simulink library "vehicle_model"  (R2020b)
settings: Solver=ode45  StartTime=0.0  StopTime=10.0  RelTol=1e-3  EnableMultiTasking=on
undefined symbols (not defined in the file): DiscIntNeverNeededParam, par_VEH, select_To_Wks_akt, stepsize, v0
libraries: $bdroot x8, pacejka_trans x6, simulink x4, body_chassis_vert x1
(part 3 of 4)

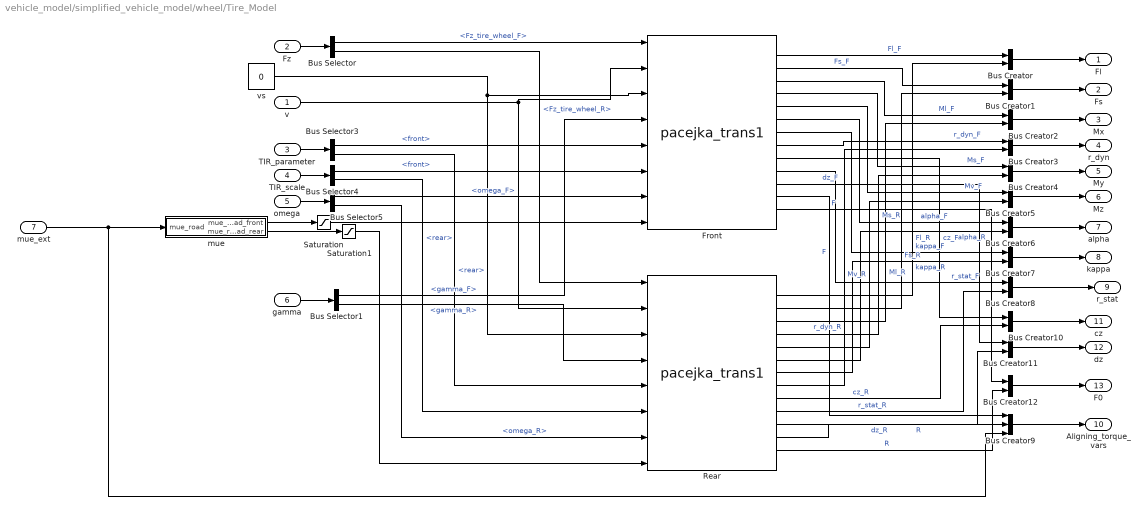
== system vehicle_model/simplified_vehicle_model/wheel/Tire_Model ==
  v : Inport
  Fz : Inport  Port=2
  TIR_parameter : Inport  Port=3
  TIR_scale : Inport  Port=4
  omega : Inport  Port=5
  gamma : Inport  Port=6
  mue_ext : Inport  Port=7
  Bus Creator{,1..8,10..12} (12 alike) : BusCreator  Inputs=2
  Bus Creator9 : BusCreator  Inputs=3
  Bus Selector : BusSelector  OutputSignals=Fz_tire_wheel_F,Fz_tire_wheel_R
  Bus Selector1 : BusSelector  OutputSignals=gamma_F,gamma_R
  Bus Selector3 : BusSelector  OutputSignals=front,rear
  Bus Selector4 : BusSelector  OutputSignals=front,rear
  Bus Selector5 : BusSelector  OutputSignals=omega_F,omega_R
  Front : pacejka_trans/pacejka_trans1  mounted_side_input=right
  Rear : pacejka_trans/pacejka_trans1  mounted_side_input=right
  Saturation : Saturate  UpperLimit=2  LowerLimit=0.05
  Saturation1 : Saturate  UpperLimit=2  LowerLimit=0.05
  mue : Subsystem
  vs : Constant  Value=0
  Fl : Outport  VectorParamsAs1DForOutWhenUnconnected=off
  Fs : Outport  Port=2  VectorParamsAs1DForOutWhenUnconnected=off
  Mx : Outport  Port=3  VectorParamsAs1DForOutWhenUnconnected=off
  r_dyn : Outport  Port=4  VectorParamsAs1DForOutWhenUnconnected=off
  My : Outport  Port=5  VectorParamsAs1DForOutWhenUnconnected=off
  Mz : Outport  Port=6  VectorParamsAs1DForOutWhenUnconnected=off
  alpha : Outport  Port=7  VectorParamsAs1DForOutWhenUnconnected=off
  kappa : Outport  Port=8  VectorParamsAs1DForOutWhenUnconnected=off
  r_stat : Outport  Port=9  VectorParamsAs1DForOutWhenUnconnected=off
  Aligning_torque_vars : Outport  Port=10  VectorParamsAs1DForOutWhenUnconnected=off
  cz : Outport  Port=11  VectorParamsAs1DForOutWhenUnconnected=off
  dz : Outport  Port=12  VectorParamsAs1DForOutWhenUnconnected=off
  F0 : Outport  Port=13  VectorParamsAs1DForOutWhenUnconnected=off
  wires:
  Front/10 -> Bus Creator8/1  "r_stat_F"
  Rear/3 -> Bus Creator2/2  "Ml_R"
  Front/8 -> Bus Creator3/1  "r_dyn_F"
  Rear/10 -> Bus Creator8/2  "r_stat_R"
  Front/5 -> Bus Creator5/1  "Mv_F"
  Bus Selector/2 -> Rear/1  "<Fz_tire_wheel_R>"
  Saturation1/1 -> Rear/8
  Bus Selector/1 -> Front/1  "<Fz_tire_wheel_F>"
  TIR_parameter/1 -> Bus Selector3/1
  Bus Selector4/1 -> Front/6  "<front>"
  Front/1 -> Bus Creator/1  "Fl_F"
  Saturation/1 -> Front/8
  Fz/1 -> Bus Selector/1
  Bus Selector4/2 -> Rear/6  "<rear>"
  Bus Selector1/1 -> Front/4  "<gamma_F>"
  Bus Selector3/1 -> Front/5  "<front>"
  omega/1 -> Bus Selector5/1
  TIR_scale/1 -> Bus Selector4/1
  Bus Selector3/2 -> Rear/5  "<rear>"
  Bus Selector5/1 -> Front/7  "<omega_F>"
  Bus Selector5/2 -> Rear/7  "<omega_R>"
  mue_ext/1 -> Bus Creator9/3, mue/1("mue_road ")
  Bus Creator1/1 -> Fs/1
  Bus Creator2/1 -> Mx/1
  Bus Creator5/1 -> Mz/1
  Rear/2 -> Bus Creator1/2  "Fs_R"
  Bus Creator12/1 -> F0/1
  Bus Creator9/1 -> Aligning_torque_vars/1
  Bus Creator/1 -> Fl/1
  Front/2 -> Bus Creator1/1  "Fs_F"
  Bus Creator6/1 -> alpha/1
  Bus Creator3/1 -> r_dyn/1
  Bus Creator7/1 -> kappa/1
  Bus Creator4/1 -> My/1
  Rear/1 -> Bus Creator/2  "Fl_R"
  Bus Creator11/1 -> dz/1
  Bus Creator10/1 -> cz/1
  Bus Creator8/1 -> r_stat/1
  Rear/9 -> Bus Creator10/2  "cz_R"
  Front/3 -> Bus Creator2/1  "Ml_F"
  Front/7 -> Bus Creator7/1  "kappa_F"
  Rear/8 -> Bus Creator3/2  "r_dyn_R"
  Rear/11 -> Bus Creator11/2  "dz_R"
  Front/11 -> Bus Creator11/1  "dz_F"
  Rear/12 -> Bus Creator9/2  "R"
  Front/13 -> Bus Creator12/1  "F"
  Front/6 -> Bus Creator6/1  "alpha_F"
  Front/12 -> Bus Creator9/1  "F"
  Front/4 -> Bus Creator4/1  "Ms_F"
  Rear/5 -> Bus Creator5/2  "Mv_R"
  Rear/6 -> Bus Creator6/2  "alpha_R"
  Rear/4 -> Bus Creator4/2  "Ms_R"
  Rear/13 -> Bus Creator12/2  "R"
  Front/9 -> Bus Creator10/1  "cz_F"
  Rear/7 -> Bus Creator7/2  "kappa_R"
  vs/1 -> Front/3, Rear/3
  v/1 -> Rear/2, Front/2
  mue/1(mue_road_front) -> Saturation/1
  mue/2(mue_road_rear) -> Saturation1/1
  gamma/1 -> Bus Selector1/1
  Bus Selector1/2 -> Rear/4  "<gamma_R>"

== system vehicle_model/simplified_vehicle_model/wheel/calc_Fz ==
  cz : Inport
  dz : Inport  Port=2
  zwheel : Inport  Port=3
  Bus Creator1 : BusCreator  Inputs=2
  Bus Selector1 : BusSelector  OutputSignals=cz_F,cz_R
  Bus Selector3 : BusSelector  OutputSignals=zwheel_F.zwheel,zwheel_R.zwheel
  Bus Selector4 : BusSelector  OutputSignals=zwheel_F.zwheelp,zwheel_R.zwheelp
  Bus Selector5 : BusSelector  OutputSignals=dz_F,dz_R
  Gain : Gain  Gain=-1
  Gain1 : Gain
  Gain2 : Gain  Gain=-1
  Gain5 : Gain
  Product{,1,4..5} (4 alike) : Product  RndMeth=Zero
  Sum4 : Sum  Inputs=|+-
  Sum5 : Sum  Inputs=|+-
  Fztire : Outport  VectorParamsAs1DForOutWhenUnconnected=off
  wires:
  Gain1/1 -> Product5/2
  Gain5/1 -> Product4/2
  Bus Selector5/2 -> Gain1/1  "<dz_R>"
  Bus Selector5/1 -> Gain5/1  "<dz_F>"
  dz/1 -> Bus Selector5/1
  Product5/1 -> Sum5/2
  Product4/1 -> Sum4/2
  Bus Selector4/1 -> Product4/1  "<zwheelp>"
  Bus Selector4/2 -> Product5/1  "<zwheelp>"
  Sum5/1 -> Bus Creator1/2  "Fz_tire_wheel_R"
  Sum4/1 -> Bus Creator1/1  "Fz_tire_wheel_F"
  Product/1 -> Sum4/1  "Fz_tire_wheel_F"
  Product1/1 -> Sum5/1  "Fz_tire_wheel_R"
  Bus Selector3/2 -> Gain2/1  "<zwheel>"
  Bus Selector3/1 -> Gain/1  "<zwheel>"
  zwheel/1 -> Bus Selector4/1, Bus Selector3/1
  Bus Creator1/1 -> Fztire/1
  Bus Selector1/2 -> Product1/1  "<cz_R>"
  cz/1 -> Bus Selector1/1
  Bus Selector1/1 -> Product/1  "<cz_F>"
  Gain/1 -> Product/2
  Gain2/1 -> Product1/2

== system vehicle_model/simplified_vehicle_model/wheel/calc_omega ==
  M_antr : Inport
  M_brems : Inport  Port=2
  r_dyn : Inport  Port=3
  My : Inport  Port=4
  Fl : Inport  Port=5
  r_stat : Inport  Port=6
  Add : Sum  Inputs=++--
  Add1 : Sum  Inputs=++--
  Add{2..7} (6 alike) : Sum
  Bus Creator : BusCreator  Inputs=2
  Bus Selector2 : BusSelector  OutputSignals=r_stat_F,r_stat_R
  Bus Selector3 : BusSelector  OutputSignals=Ms_F,Ms_R
  Bus Selector4 : BusSelector  OutputSignals=Fl_F,Fl_R
  Bus Selector6 : BusSelector  OutputSignals=r_dyn_F,r_dyn_R
  Bus Selector7 : BusSelector  OutputSignals=M_antr_RF,M_antr_LF,M_antr_RR,M_antr_LR
  Bus Selector8 : BusSelector  OutputSignals=M_brems_RF,M_brems_LF,M_brems_RR,M_brems_LR
  Constant : Constant  Value=v0
  Discrete-Time Integrator1 : DiscreteIntegrator  ExternalReset=sampled level  InitialConditionSource=external  InitialCondition=v0/0.3  SampleTime=-1  ICPrevOutput=DiscIntNeverNeededParam  ICPrevScaledInput=DiscIntNeverNeededParam
  Discrete-Time Integrator2 : DiscreteIntegrator  ExternalReset=sampled level  InitialConditionSource=external  InitialCondition=v0/0.3  SampleTime=-1  ICPrevOutput=DiscIntNeverNeededParam  ICPrevScaledInput=DiscIntNeverNeededParam
  Divide{,1,4..5} (4 alike) : Product  Inputs=*/
  Gain{,1..3} (4 alike) : Gain  Gain=0.5
  Product4 : Product  RndMeth=Zero
  Product5 : Product  RndMeth=Zero
  Unit Delay1 : UnitDelay  InitialCondition=par_VEH.r_stat0  SampleTime=-1  HasFrameUpgradeWarning=on
  Unit Delay2 : UnitDelay  InitialCondition=par_VEH.r_stat0  SampleTime=-1  HasFrameUpgradeWarning=on
  friction : Subsystem
  omega : Outport  VectorParamsAs1DForOutWhenUnconnected=off
  wires:
  friction/2(M_fric_R) -> Add1/4
  friction/1(M_fric_F) -> Add/4
  Bus Selector6/2 -> Unit Delay2/1  "<r_dyn_R>"
  Bus Selector6/1 -> Unit Delay1/1  "<r_dyn_F>"
  r_dyn/1 -> Bus Selector6/1
  Gain3/1 -> Add5/2  "M_brems_R"
  Gain1/1 -> Add5/1  "M_antr_R"
  Gain2/1 -> Add4/2  "M_brems_F"
  Gain/1 -> Add4/1  "M_antr_F"
  [Iwf] -> Divide/2
  Unit Delay2/1 -> Divide5/2
  Unit Delay1/1 -> Divide4/2
  Divide5/1 -> Discrete-Time Integrator1/3
  Divide4/1 -> Discrete-Time Integrator2/3
  Constant/1 -> Divide5/1, Divide4/1
  Divide1/1 -> Discrete-Time Integrator1/1  "omegap_R"
  Divide/1 -> Discrete-Time Integrator2/1  "omegap_F"
  Bus Selector3/2 -> Add1/1  "<Ms_R>"
  Bus Selector3/1 -> Add/1  "<Ms_F>"
  Fl/1 -> Bus Selector4/1
  My/1 -> Bus Selector3/1
  r_stat/1 -> Bus Selector2/1
  Add/1 -> Divide/1
  Add1/1 -> Divide1/1
  Add4/1 -> Add/2
  Add5/1 -> Add1/2
  Bus Selector4/1 -> Product4/1  "<Fl_F>"
  Bus Selector2/1 -> Product4/2  "<r_stat_F>"
  Bus Selector4/2 -> Product5/1  "<Fl_R>"
  Bus Selector2/2 -> Product5/2  "<r_stat_R>"
  Product4/1 -> Add/3
  Product5/1 -> Add1/3
  Bus Creator/1 -> friction/1(omega), omega/1
  Discrete-Time Integrator2/1 -> Bus Creator/1  "omega_F"
  Discrete-Time Integrator1/1 -> Bus Creator/2  "omega_R"
  [Iwr] -> Divide1/2
  [reset] -> Discrete-Time Integrator2/2, Discrete-Time Integrator1/2
  Bus Selector7/3 -> Add3/1  "<M_antr_RR>"
  Bus Selector8/3 -> Add7/1  "<M_brems_RR>"
  Bus Selector7/4 -> Add3/2  "<M_antr_LR>"
  Bus Selector8/4 -> Add7/2  "<M_brems_LR>"
  Bus Selector7/2 -> Add2/2  "<M_antr_LF>"
  Bus Selector8/1 -> Add6/1  "<M_brems_RF>"
  Bus Selector7/1 -> Add2/1  "<M_antr_RF>"
  M_brems/1 -> Bus Selector8/1
  M_antr/1 -> Bus Selector7/1
  Bus Selector8/2 -> Add6/2  "<M_brems_LF>"
  Add2/1 -> Gain/1
  Add3/1 -> Gain1/1
  Add6/1 -> Gain2/1
  Add7/1 -> Gain3/1

== system vehicle_model/simplified_vehicle_model/wheel/v0_korr ==
  vl : Inport
  r_dyn : Inport  Port=2
  omega : Inport  Port=3
  Bus Creator : BusCreator  Inputs=2
  Bus Selector1 : BusSelector  OutputSignals=r_dyn_F,r_dyn_R
  Bus Selector2 : BusSelector  OutputSignals=omega_F,omega_R
  Subsystem1 : Subsystem
  Subsystem2 : $bdroot/vehicle_model/wheel/v0_korr/Subsystem4  SystemSampleTime=-1  VariantActivationTime=update diagram  Latency=0  AutoFrameSizeCalculation=off
  v_low : Constant  Value=0.01  VectorParams1D=off
  omega_out : Outport  VectorParamsAs1DForOutWhenUnconnected=off
  wires:
  r_dyn/1 -> Bus Selector1/1
  omega/1 -> Bus Selector2/1
  Bus Creator/1 -> omega_out/1
  v_low/1 -> Subsystem1/2(v_low), Subsystem2/2
  Bus Selector1/1 -> Subsystem1/3(r_dyn)  "<r_dyn_F>"
  Bus Selector1/2 -> Subsystem2/3  "<r_dyn_R>"
  Bus Selector2/1 -> Subsystem1/4(omega)  "<omega_F>"
  Bus Selector2/2 -> Subsystem2/4  "<omega_R>"
  Subsystem1/1(omega_out) -> Bus Creator/1  "omega_F"
  Subsystem2/1 -> Bus Creator/2  "omega_R"
  vl/1 -> Subsystem2/1, Subsystem1/1(vl)

== system vehicle_model/simplified_vehicle_model/wheel/wheel_lift ==
  Fz_spring : Inport
  Fz_tire_wheel : Inport  Port=2
  init_pos : Inport  Port=3
  Bus Selector : BusSelector  OutputSignals=Fz_tire_wheel_F,Fz_tire_wheel_R
  Bus Selector1 : BusSelector  OutputSignals=Fz_Front,Fz_Rear
  wheel_lift_F : Subsystem
  wheel_lift_R : Subsystem
  zroad : Subsystem
  zwheel_F : Outport  VectorParamsAs1DForOutWhenUnconnected=off
  zwheel_R : Outport  Port=2  VectorParamsAs1DForOutWhenUnconnected=off
  wires:
  zroad/2(zroad_rear) -> wheel_lift_R/3(z_init_rear)
  zroad/1(zroad_front) -> wheel_lift_F/3(z_init_front)
  init_pos/1 -> zroad/1(init_pos)
  Bus Selector1/1 -> wheel_lift_F/2(Fzt)  "<Fz_Front>"
  Bus Selector1/2 -> wheel_lift_R/2(Fzt)  "<Fz_Rear>"
  Bus Selector/2 -> wheel_lift_R/1(Fz_tire_wheel)  "<Fz_tire_wheel_R>"
  Bus Selector/1 -> wheel_lift_F/1(Fz_tire_wheel)  "<Fz_tire_wheel_F>"
  Fz_spring/1 -> Bus Selector1/1
  wheel_lift_R/1(zwheel_rear) -> zwheel_R/1
  Fz_tire_wheel/1 -> Bus Selector/1
  wheel_lift_F/1(zwheel_front) -> zwheel_F/1

== system vehicle_model/vehicle_model/Transformation/trafo_matrix ==
  psi : Inport
  theta : Inport  Port=2
  phi : Inport  Port=3
  Add{1..4} (4 alike) : Sum
  Matrix Concatenate : Concatenate  NumInputs=3  Mode=Multidimensional array  ConcatenateDimension=2
  Matrix Concatenate1 : Concatenate  NumInputs=3
  Matrix Concatenate2 : Concatenate  NumInputs=3
  Matrix Concatenate3 : Concatenate  NumInputs=3
  Product{,1,3,5..6,8,10..11} (8 alike) : Product
  Product{2,4,7,9} (4 alike) : Product  Inputs=3
  Trigonometric Function : Trigonometry  Operator=cos
  Trigonometric Function2 : Trigonometry  Operator=cos
  Trigonometric Function3 : Trigonometry  Operator=cos
  Trigonometric Function6 : Trigonometry
  Trigonometric Function7 : Trigonometry
  Trigonometric Function8 : Trigonometry
  Unary Minus : UnaryMinus
  Unary Minus1 : UnaryMinus
  Unary Minus2 : UnaryMinus
  OT3 : Outport  VectorParamsAs1DForOutWhenUnconnected=off
  wires:
  Product11/1 -> Matrix Concatenate3/2
  Product1/1 -> Add1/1
  Trigonometric Function8/1 -> Unary Minus2/1, Product9/2, Product7/2, Product4/2, Product2/2
  Product4/1 -> Add2/2
  Matrix Concatenate/1 -> OT3/1
  Add2/1 -> Matrix Concatenate1/3
  Trigonometric Function6/1 -> Product3/2, Product2/3, Product11/2, Product8/2, Product7/3
  Trigonometric Function/1 -> Product/1, Unary Minus1/1, Product6/1, Product4/1, Product2/1
  Trigonometric Function2/1 -> Product/2, Product5/2, Product10/1, Product11/1
  Trigonometric Function7/1 -> Unary Minus/1, Product9/1, Product7/1, Product5/1, Product3/1
  Product/1 -> Matrix Concatenate1/1
  Product5/1 -> Matrix Concatenate2/1
  Unary Minus/1 -> Product1/1
  Product3/1 -> Add2/1
  Trigonometric Function3/1 -> Product1/2, Product4/3, Product6/2, Product9/3, Product10/2
  Add1/1 -> Matrix Concatenate1/2
  Unary Minus1/1 -> Product8/1
  Product7/1 -> Add3/2
  theta/1 -> Trigonometric Function8/1, Trigonometric Function2/1
  psi/1 -> Trigonometric Function/1, Trigonometric Function7/1
  Add3/1 -> Matrix Concatenate2/2
  Product8/1 -> Add4/1
  Product9/1 -> Add4/2
  phi/1 -> Trigonometric Function3/1, Trigonometric Function6/1
  Product6/1 -> Add3/1
  Matrix Concatenate3/1 -> Matrix Concatenate/3
  Matrix Concatenate2/1 -> Matrix Concatenate/2
  Unary Minus2/1 -> Matrix Concatenate3/1
  Product10/1 -> Matrix Concatenate3/3
  Add4/1 -> Matrix Concatenate2/3
  Matrix Concatenate1/1 -> Matrix Concatenate/1
  Product2/1 -> Add1/2

== system vehicle_model/vehicle_model/Transformation/trafo_matrix1 ==
  psi : Inport
  theta : Inport  Port=2
  Constant : Constant  Value=0
  Constant1 : Constant  Value=0
  Constant2 : Constant
  Constant3 : Constant  Value=0
  Matrix Concatenate : Concatenate  NumInputs=3  Mode=Multidimensional array  ConcatenateDimension=2
  Matrix Concatenate1 : Concatenate  NumInputs=3
  Matrix Concatenate2 : Concatenate  NumInputs=3
  Matrix Concatenate3 : Concatenate  NumInputs=3
  Product3 : Product
  Product6 : Product
  Trigonometric Function : Trigonometry  Operator=cos
  Trigonometric Function2 : Trigonometry  Operator=cos
  Trigonometric Function7 : Trigonometry
  Trigonometric Function8 : Trigonometry
  Unary Minus : UnaryMinus
  Unary Minus1 : UnaryMinus
  OTo : Outport  VectorParamsAs1DForOutWhenUnconnected=off
  wires:
  Unary Minus1/1 -> Matrix Concatenate3/3
  Trigonometric Function8/1 -> Unary Minus1/1
  Constant3/1 -> Matrix Concatenate3/2
  Constant2/1 -> Matrix Concatenate3/1
  Constant1/1 -> Matrix Concatenate2/1
  Constant/1 -> Matrix Concatenate1/1
  Matrix Concatenate1/1 -> Matrix Concatenate/1
  Matrix Concatenate2/1 -> Matrix Concatenate/2
  Matrix Concatenate3/1 -> Matrix Concatenate/3
  Product6/1 -> Matrix Concatenate2/3
  psi/1 -> Trigonometric Function7/1, Trigonometric Function/1
  theta/1 -> Trigonometric Function8/1, Trigonometric Function2/1
  Unary Minus/1 -> Matrix Concatenate1/2
  Trigonometric Function7/1 -> Product6/2, Unary Minus/1
  Trigonometric Function2/1 -> Product6/1, Product3/2
  Trigonometric Function/1 -> Matrix Concatenate2/2, Product3/1
  Product3/1 -> Matrix Concatenate1/3
  Matrix Concatenate/1 -> OTo/1

== system vehicle_model/vehicle_model/Transformation1/trafo_matrix ==
  psi : Inport
  theta : Inport  Port=2
  phi : Inport  Port=3
  Add{1..4} (4 alike) : Sum
  Matrix Concatenate : Concatenate  NumInputs=3  Mode=Multidimensional array  ConcatenateDimension=2
  Matrix Concatenate1 : Concatenate  NumInputs=3
  Matrix Concatenate2 : Concatenate  NumInputs=3
  Matrix Concatenate3 : Concatenate  NumInputs=3
  Product{,1..2,5..8,10} (8 alike) : Product
  Product{3..4,9,12} (4 alike) : Product  Inputs=3
  Trigonometric Function : Trigonometry  Operator=cos
  Trigonometric Function2 : Trigonometry  Operator=cos
  Trigonometric Function3 : Trigonometry  Operator=cos
  Trigonometric Function6 : Trigonometry
  Trigonometric Function7 : Trigonometry
  Trigonometric Function8 : Trigonometry
  Unary Minus1 : UnaryMinus
  Unary Minus3 : UnaryMinus
  Unary Minus4 : UnaryMinus
  OT3 : Outport  VectorParamsAs1DForOutWhenUnconnected=off
  wires:
  Product10/1 -> Matrix Concatenate3/3
  Add4/1 -> Matrix Concatenate3/2
  Product9/1 -> Add4/2
  Product8/1 -> Add4/1
  Unary Minus1/1 -> Product8/1
  Add3/1 -> Matrix Concatenate3/1
  Product12/1 -> Add3/2
  Product7/1 -> Add3/1
  Add2/1 -> Matrix Concatenate2/2
  Product4/1 -> Add2/2
  Product5/1 -> Add2/1
  Add1/1 -> Matrix Concatenate2/1
  Product3/1 -> Add1/2
  Product2/1 -> Add1/1
  Unary Minus4/1 -> Product2/1
  Trigonometric Function8/1 -> Unary Minus3/1, Product3/2, Product4/2, Product12/2, Product9/2
  Matrix Concatenate/1 -> OT3/1
  Unary Minus3/1 -> Matrix Concatenate1/3
  Trigonometric Function6/1 -> Product3/3, Product4/3, Product6/2, Product7/2, Product8/2
  Trigonometric Function/1 -> Product/1, Product3/1, Product5/1, Product12/1, Unary Minus1/1
  Trigonometric Function2/1 -> Product/2, Product1/2, Product6/1, Product10/1
  Product/1 -> Matrix Concatenate1/1
  Trigonometric Function7/1 -> Product1/1, Unary Minus4/1, Product4/1, Product7/1, Product9/1
  Trigonometric Function3/1 -> Product2/2, Product5/2, Product12/3, Product9/3, Product10/2
  Product1/1 -> Matrix Concatenate1/2
  theta/1 -> Trigonometric Function2/1, Trigonometric Function8/1
  psi/1 -> Trigonometric Function/1, Trigonometric Function7/1
  phi/1 -> Trigonometric Function3/1, Trigonometric Function6/1
  Product6/1 -> Matrix Concatenate2/3
  Matrix Concatenate3/1 -> Matrix Concatenate/3
  Matrix Concatenate2/1 -> Matrix Concatenate/2
  Matrix Concatenate1/1 -> Matrix Concatenate/1

== system vehicle_model/vehicle_model/calc_init/pitch ==
  init_pos : Inport
  Add : Sum
  Add1 : Sum
  Add2 : Sum  Inputs=+-
  Bus Selector : BusSelector  OutputSignals=zroad_RF0,zroad_LF0,zroad_RR0,zroad_LR0
  Divide : Product  Inputs=*/
  Gain : Gain  Gain=0.5
  Gain1 : Gain  Gain=0.5
  Trigonometric Function : Trigonometry  Operator=atan
  init_theta : Outport  VectorParamsAs1DForOutWhenUnconnected=off
  wires:
  Bus Selector/3 -> Add1/1  "<zroad_RR0>"
  Bus Selector/2 -> Add/2  "<zroad_LF0>"
  init_pos/1 -> Bus Selector/1
  Bus Selector/1 -> Add/1  "<zroad_RF0>"
  Add/1 -> Gain/1
  Add1/1 -> Gain1/1
  Bus Selector/4 -> Add1/2  "<zroad_LR0>"
  Gain/1 -> Add2/1
  Gain1/1 -> Add2/2
  Add2/1 -> Divide/1
  Divide/1 -> Trigonometric Function/1
  [l] -> Divide/2
  Trigonometric Function/1 -> init_theta/1

== system vehicle_model/vehicle_model/calc_init/roll ==
  init_pos : Inport
  Add : Sum
  Add1 : Sum
  Add2 : Sum  Inputs=+-
  Add3 : Sum
  Bus Selector : BusSelector  OutputSignals=zroad_RF0,zroad_RR0,zroad_LF0,zroad_LR0
  Divide : Product  Inputs=*/
  Gain : Gain  Gain=0.5
  Gain1 : Gain  Gain=0.5
  Gain2 : Gain  Gain=0.5
  Trigonometric Function : Trigonometry  Operator=atan
  init_phi : Outport  VectorParamsAs1DForOutWhenUnconnected=off
  wires:
  Trigonometric Function/1 -> init_phi/1
  Gain2/1 -> Divide/2
  Add3/1 -> Gain2/1
  [sR] -> Add3/2
  [sF] -> Add3/1
  Divide/1 -> Trigonometric Function/1
  Add2/1 -> Divide/1
  Gain1/1 -> Add2/2
  Gain/1 -> Add2/1
  Bus Selector/2 -> Add/2  "<zroad_RR0>"
  Bus Selector/4 -> Add1/2  "<zroad_LR0>"
  Add1/1 -> Gain1/1
  Add/1 -> Gain/1
  Bus Selector/3 -> Add1/1  "<zroad_LF0>"
  Bus Selector/1 -> Add/1  "<zroad_RF0>"
  init_pos/1 -> Bus Selector/1

== system vehicle_model/vehicle_model/calc_init/vertical ==
  init_pos : Inport
  theta : Inport  Port=2
  Add : Sum
  Add1 : Sum
  Bus Selector : BusSelector  OutputSignals=zroad_RF0,zroad_LF0
  Gain : Gain  Gain=0.5
  Product : Product  RndMeth=Zero
  Trigonometric Function : Trigonometry
  init_z0 : Outport  VectorParamsAs1DForOutWhenUnconnected=off
  wires:
  Add1/1 -> init_z0/1
  Product/1 -> Add1/2
  Trigonometric Function/1 -> Product/2
  theta/1 -> Trigonometric Function/1
  [lF] -> Product/1
  Gain/1 -> Add1/1
  Add/1 -> Gain/1
  Bus Selector/2 -> Add/2  "<zroad_LF0>"
  Bus Selector/1 -> Add/1  "<zroad_RF0>"
  init_pos/1 -> Bus Selector/1

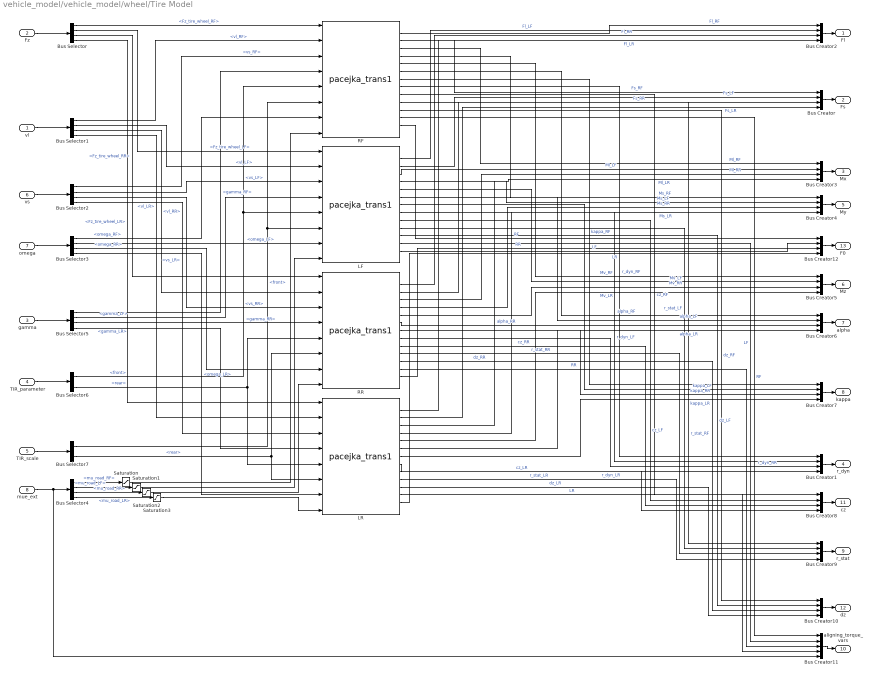
== system vehicle_model/vehicle_model/wheel/Tire Model ==
  vl : Inport
  Fz : Inport  Port=2
  gamma : Inport  Port=3
  TIR_parameter : Inport  Port=4
  TIR_scale : Inport  Port=5
  vs : Inport  Port=6
  omega : Inport  Port=7
  mue_ext : Inport  Port=8
  Bus Creator{,1..10,12} (12 alike) : BusCreator  Inputs=4
  Bus Creator11 : BusCreator  Inputs=5
  Bus Selector : BusSelector  OutputSignals=Fz_tire_wheel_RF,Fz_tire_wheel_LF,Fz_tire_wheel_RR,Fz_tire_wheel_LR
  Bus Selector1 : BusSelector  OutputSignals=vl_RF,vl_LF,vl_RR,vl_LR
  Bus Selector2 : BusSelector  OutputSignals=vs_RF,vs_LF,vs_RR,vs_LR
  Bus Selector3 : BusSelector  OutputSignals=omega_RF,omega_LF,omega_RR,omega_LR
  Bus Selector4 : BusSelector  OutputSignals=mu_road_RF,mu_road_LF,mu_road_RR,mu_road_LR
  Bus Selector5 : BusSelector  OutputSignals=gamma_RF,gamma_LF,gamma_RR,gamma_LR
  Bus Selector6 : BusSelector  OutputSignals=front,rear
  Bus Selector7 : BusSelector  OutputSignals=front,rear
  LF : pacejka_trans/pacejka_trans1  mounted_side_input=left
  LR : pacejka_trans/pacejka_trans1  mounted_side_input=left
  RF : pacejka_trans/pacejka_trans1  mounted_side_input=right
  RR : pacejka_trans/pacejka_trans1  mounted_side_input=right
  Saturation{,1..3} (4 alike) : Saturate  UpperLimit=2  LowerLimit=0.05
  Fl : Outport  VectorParamsAs1DForOutWhenUnconnected=off
  Fs : Outport  Port=2  VectorParamsAs1DForOutWhenUnconnected=off
  Mx : Outport  Port=3  VectorParamsAs1DForOutWhenUnconnected=off
  r_dyn : Outport  Port=4  VectorParamsAs1DForOutWhenUnconnected=off
  My : Outport  Port=5  VectorParamsAs1DForOutWhenUnconnected=off
  Mz : Outport  Port=6  VectorParamsAs1DForOutWhenUnconnected=off
  alpha : Outport  Port=7  VectorParamsAs1DForOutWhenUnconnected=off
  kappa : Outport  Port=8  VectorParamsAs1DForOutWhenUnconnected=off
  r_stat : Outport  Port=9  VectorParamsAs1DForOutWhenUnconnected=off
  aligning_torque_vars : Outport  Port=10  VectorParamsAs1DForOutWhenUnconnected=off
  cz : Outport  Port=11  VectorParamsAs1DForOutWhenUnconnected=off
  dz : Outport  Port=12  VectorParamsAs1DForOutWhenUnconnected=off
  F0 : Outport  Port=13  VectorParamsAs1DForOutWhenUnconnected=off
  wires:
  LR/13 -> Bus Creator12/4  "LR"
  RR/13 -> Bus Creator12/3  "RR"
  LF/13 -> Bus Creator12/2  "LF"
  RF/13 -> Bus Creator12/1  "RF"
  Bus Creator12/1 -> F0/1
  LR/12 -> Bus Creator11/4  "LR"
  RR/12 -> Bus Creator11/3  "RR"
  LF/12 -> Bus Creator11/2  "LF"
  RF/12 -> Bus Creator11/1  "RF"
  Bus Creator11/1 -> aligning_torque_vars/1
  Bus Selector7/2 -> RR/6, LR/6  "<rear>"
  Bus Selector6/2 -> LR/5, RR/5  "<rear>"
  Bus Selector7/1 -> RF/6, LF/6  "<front>"
  Bus Selector6/1 -> LF/5, RF/5  "<front>"
  TIR_scale/1 -> Bus Selector7/1
  TIR_parameter/1 -> Bus Selector6/1
  Saturation3/1 -> LR/8
  Saturation2/1 -> RR/8
  Saturation1/1 -> LF/8
  Saturation/1 -> RF/8
  Bus Selector5/4 -> LR/4  "<gamma_LR>"
  Bus Selector5/3 -> RR/4  "<gamma_RR>"
  Bus Selector5/2 -> LF/4  "<gamma_LF>"
  Bus Selector5/1 -> RF/4  "<gamma_RF>"
  gamma/1 -> Bus Selector5/1
  LR/11 -> Bus Creator10/4  "dz_LR"
  RR/11 -> Bus Creator10/3  "dz_RR"
  LF/11 -> Bus Creator10/2  "dz_LF"
  RF/11 -> Bus Creator10/1  "dz_RF"
  Bus Creator10/1 -> dz/1
  LR/10 -> Bus Creator9/4  "r_stat_LR"
  RR/10 -> Bus Creator9/3  "r_stat_RR"
  LF/10 -> Bus Creator9/2  "r_stat_LF"
  RF/10 -> Bus Creator9/1  "r_stat_RF"
  Bus Creator9/1 -> r_stat/1
  LR/9 -> Bus Creator8/4  "cz_LR"
  RR/9 -> Bus Creator8/3  "cz_RR"
  LF/9 -> Bus Creator8/2  "cz_LF"
  RF/9 -> Bus Creator8/1  "cz_RF"
  Bus Creator8/1 -> cz/1
  Bus Selector4/4 -> Saturation3/1  "<mu_road_LR>"
  Bus Selector4/3 -> Saturation2/1  "<mu_road_RR>"
  Bus Selector4/2 -> Saturation1/1  "<mu_road_LF>"
  Bus Selector4/1 -> Saturation/1  "<mu_road_RF>"
  mue_ext/1 -> Bus Selector4/1, Bus Creator11/5
  Bus Creator/1 -> Fs/1
  RF/2 -> Bus Creator/1  "Fs_RF"
  LF/2 -> Bus Creator/2  "Fs_LF"
  LR/2 -> Bus Creator/4  "Fs_LR"
  RR/2 -> Bus Creator/3  "Fs_RR"
  Bus Creator1/1 -> r_dyn/1
  RF/8 -> Bus Creator1/1  "r_dyn_RF"
  LF/8 -> Bus Creator1/2  "r_dyn_LF"
  RR/8 -> Bus Creator1/3  "r_dyn_RR"
  LR/8 -> Bus Creator1/4  "r_dyn_LR"
  Bus Creator2/1 -> Fl/1
  RF/1 -> Bus Creator2/1  "Fl_RF"
  LF/1 -> Bus Creator2/2  "Fl_LF"
  RR/1 -> Bus Creator2/3  "Fl_RR"
  LR/1 -> Bus Creator2/4  "Fl_LR"
  Bus Creator3/1 -> Mx/1
  Bus Creator4/1 -> My/1
  Bus Creator5/1 -> Mz/1
  Bus Creator6/1 -> alpha/1
  Bus Creator7/1 -> kappa/1
  RF/3 -> Bus Creator3/1  "Ml_RF"
  LF/3 -> Bus Creator3/2  "Ml_LF"
  RR/3 -> Bus Creator3/3  "Ml_RR"
  LR/3 -> Bus Creator3/4  "Ml_LR"
  RF/4 -> Bus Creator4/1  "Ms_RF"
  LF/4 -> Bus Creator4/2  "Ms_LF"
  RR/4 -> Bus Creator4/3  "Ms_RR"
  LR/4 -> Bus Creator4/4  "Ms_LR"
  RF/5 -> Bus Creator5/1  "Mv_RF"
  LF/5 -> Bus Creator5/2  "Mv_LF"
  RR/5 -> Bus Creator5/3  "Mv_RR"
  LR/5 -> Bus Creator5/4  "Mv_LR"
  RF/6 -> Bus Creator6/1  "alpha_RF"
  RR/6 -> Bus Creator6/3  "alpha_RR"
  LF/6 -> Bus Creator6/2  "alpha_LF"
  LR/6 -> Bus Creator6/4  "alpha_LR"
  RF/7 -> Bus Creator7/1  "kappa_RF"
  LF/7 -> Bus Creator7/2  "kappa_LF"
  RR/7 -> Bus Creator7/3  "kappa_RR"
  LR/7 -> Bus Creator7/4  "kappa_LR"
  Fz/1 -> Bus Selector/1
  vl/1 -> Bus Selector1/1
  vs/1 -> Bus Selector2/1
  Bus Selector/1 -> RF/1  "<Fz_tire_wheel_RF>"
  Bus Selector/2 -> LF/1  "<Fz_tire_wheel_LF>"
  Bus Selector/3 -> RR/1  "<Fz_tire_wheel_RR>"
  Bus Selector/4 -> LR/1  "<Fz_tire_wheel_LR>"
  Bus Selector1/1 -> RF/2  "<vl_RF>"
  Bus Selector1/2 -> LF/2  "<vl_LF>"
  Bus Selector1/3 -> RR/2  "<vl_RR>"
  Bus Selector1/4 -> LR/2  "<vl_LR>"
  omega/1 -> Bus Selector3/1
  Bus Selector3/1 -> RF/7  "<omega_RF>"
  Bus Selector3/2 -> LF/7  "<omega_LF>"
  Bus Selector3/3 -> RR/7  "<omega_RR>"
  Bus Selector3/4 -> LR/7  "<omega_LR>"
  Bus Selector2/1 -> RF/3  "<vs_RF>"
  Bus Selector2/2 -> LF/3  "<vs_LF>"
  Bus Selector2/3 -> RR/3  "<vs_RR>"
  Bus Selector2/4 -> LR/3  "<vs_LR>"

== system vehicle_model/vehicle_model/wheel/calc_Fz ==
  cz : Inport
  dz : Inport  Port=2
  zwheel : Inport  Port=3
  Bus Creator : BusCreator  Inputs=4
  Bus Selector : BusSelector  OutputSignals=cz_RF,cz_LF,cz_RR,cz_LR
  Bus Selector2 : BusSelector  OutputSignals=zwheel_RF.zwheel,zwheel_LF.zwheel,zwheel_RR.zwheel,zwheel_LR.zwheel
  Bus Selector3 : BusSelector  OutputSignals=dz_RF,dz_LF,dz_RR,dz_LR
  Bus Selector4 : BusSelector  OutputSignals=zwheel_RF.zwheelp,zwheel_LF.zwheelp,zwheel_RR.zwheelp,zwheel_LR.zwheelp
  Gain{,4,6..7} (4 alike) : Gain  Gain=-1
  Gain{1..3,5} (4 alike) : Gain
  Product{,1..7} (8 alike) : Product  RndMeth=Zero
  Sum{4..7} (4 alike) : Sum  Inputs=|+-
  Fztire : Outport  VectorParamsAs1DForOutWhenUnconnected=off
  wires:
  Bus Selector/1 -> Product/1  "<cz_RF>"
  cz/1 -> Bus Selector/1
  Bus Selector/2 -> Product1/1  "<cz_LF>"
  Bus Creator/1 -> Fztire/1
  zwheel/1 -> Bus Selector2/1, Bus Selector4/1
  Bus Selector2/1 -> Gain4/1  "<zwheel>"
  Bus Selector2/2 -> Gain6/1  "<zwheel>"
  Bus Selector2/3 -> Gain/1  "<zwheel>"
  Bus Selector2/4 -> Gain7/1  "<zwheel>"
  Bus Selector/3 -> Product2/1  "<cz_RR>"
  Bus Selector/4 -> Product3/1  "<cz_LR>"
  Product3/1 -> Sum7/1  "Fz_tire_wheel_LR"
  Product2/1 -> Sum6/1  "Fz_tire_wheel_RR"
  Product1/1 -> Sum5/1  "Fz_tire_wheel_LF"
  Product/1 -> Sum4/1  "Fz_tire_wheel_RF"
  Sum4/1 -> Bus Creator/1  "Fz_tire_wheel_RF"
  Sum5/1 -> Bus Creator/2  "Fz_tire_wheel_LF"
  Sum6/1 -> Bus Creator/3  "Fz_tire_wheel_RR"
  Sum7/1 -> Bus Creator/4  "Fz_tire_wheel_LR"
  Bus Selector4/4 -> Product7/1  "<zwheelp>"
  Bus Selector4/3 -> Product6/1  "<zwheelp>"
  Bus Selector4/2 -> Product5/1  "<zwheelp>"
  Bus Selector4/1 -> Product4/1  "<zwheelp>"
  Product4/1 -> Sum4/2
  Product5/1 -> Sum5/2
  Product6/1 -> Sum6/2
  Product7/1 -> Sum7/2
  dz/1 -> Bus Selector3/1
  Bus Selector3/1 -> Gain5/1  "<dz_RF>"
  Bus Selector3/2 -> Gain1/1  "<dz_LF>"
  Bus Selector3/3 -> Gain2/1  "<dz_RR>"
  Bus Selector3/4 -> Gain3/1  "<dz_LR>"
  Gain5/1 -> Product4/2
  Gain1/1 -> Product5/2
  Gain2/1 -> Product6/2
  Gain3/1 -> Product7/2
  Gain/1 -> Product2/2
  Gain4/1 -> Product/2
  Gain6/1 -> Product1/2
  Gain7/1 -> Product3/2

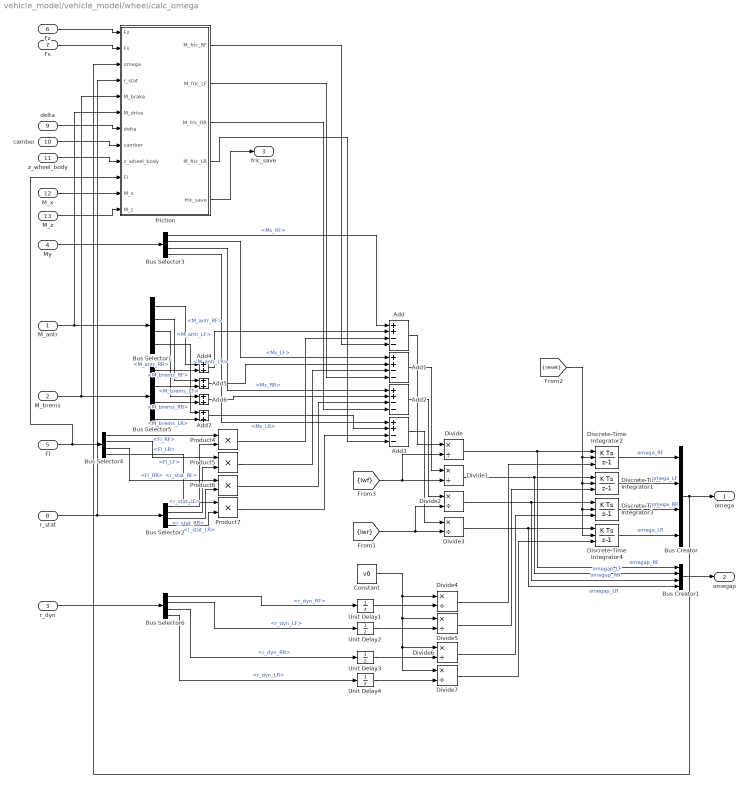
== system vehicle_model/vehicle_model/wheel/calc_omega ==
  M_antr : Inport
  M_brems : Inport  Port=2
  r_dyn : Inport  Port=3
  My : Inport  Port=4
  Fl : Inport  Port=5
  Fz : Inport  Port=6
  Fs : Inport  Port=7
  r_stat : Inport  Port=8
  delta : Inport  Port=9
  camber : Inport  Port=10
  z_wheel_body : Inport  Port=11
  M_x : Inport  Port=12
  M_z : Inport  Port=13
  Add{,1..3} (4 alike) : Sum  Inputs=++--
  Add{4..7} (4 alike) : Sum
  Bus Creator : BusCreator  Inputs=4
  Bus Creator1 : BusCreator  Inputs=4
  Bus Selector1 : BusSelector  OutputSignals=M_antr_RF,M_antr_LF,M_antr_RR,M_antr_LR
  Bus Selector2 : BusSelector  OutputSignals=r_stat_RF,r_stat_LF,r_stat_RR,r_stat_LR
  Bus Selector3 : BusSelector  OutputSignals=Ms_RF,Ms_LF,Ms_RR,Ms_LR
  Bus Selector4 : BusSelector  OutputSignals=Fl_RF,Fl_LF,Fl_RR,Fl_LR
  Bus Selector5 : BusSelector  OutputSignals=M_brems_RF,M_brems_LF,M_brems_RR,M_brems_LR
  Bus Selector6 : BusSelector  OutputSignals=r_dyn_RF,r_dyn_LF,r_dyn_RR,r_dyn_LR
  Constant : Constant  Value=v0
  Discrete-Time Integrator{1..4} (4 alike) : DiscreteIntegrator  ExternalReset=sampled level  InitialConditionSource=external  InitialCondition=v0/0.3  SampleTime=-1  ICPrevOutput=DiscIntNeverNeededParam  ICPrevScaledInput=DiscIntNeverNeededParam
  Divide{,1..7} (8 alike) : Product  Inputs=*/
  Product{4..7} (4 alike) : Product  RndMeth=Zero
  Unit Delay{1..4} (4 alike) : UnitDelay  InitialCondition=par_VEH.r_stat0  SampleTime=-1  HasFrameUpgradeWarning=on
  friction : Subsystem
  omega : Outport  VectorParamsAs1DForOutWhenUnconnected=off
  omegap : Outport  Port=2  VectorParamsAs1DForOutWhenUnconnected=off
  fric_save : Outport  Port=3  VectorParamsAs1DForOutWhenUnconnected=off
  wires:
  [reset] -> Discrete-Time Integrator4/2, Discrete-Time Integrator3/2, Discrete-Time Integrator1/2, Discrete-Time Integrator2/2
  [Iwr] -> Divide2/2, Divide3/2
  Discrete-Time Integrator4/1 -> Bus Creator/4  "omega_LR"
  Discrete-Time Integrator3/1 -> Bus Creator/3  "omega_RR"
  Discrete-Time Integrator1/1 -> Bus Creator/2  "omega_LF"
  Discrete-Time Integrator2/1 -> Bus Creator/1  "omega_RF"
  Bus Creator1/1 -> omegap/1
  Bus Creator/1 -> omega/1, friction/3(omega)
  Product6/1 -> Add2/3
  Product5/1 -> Add1/3
  Product4/1 -> Add/3
  Bus Selector2/4 -> Product7/2  "<r_stat_LR>"
  Bus Selector4/4 -> Product7/1  "<Fl_LR>"
  Bus Selector2/3 -> Product6/2  "<r_stat_RR>"
  Bus Selector4/3 -> Product6/1  "<Fl_RR>"
  Bus Selector2/2 -> Product5/2  "<r_stat_LF>"
  Bus Selector4/2 -> Product5/1  "<Fl_LF>"
  Bus Selector2/1 -> Product4/2  "<r_stat_RF>"
  Bus Selector4/1 -> Product4/1  "<Fl_RF>"
  Add7/1 -> Add3/2
  Add6/1 -> Add2/2
  Add5/1 -> Add1/2
  Add4/1 -> Add/2
  Add3/1 -> Divide3/1
  Add2/1 -> Divide2/1
  Add1/1 -> Divide1/1
  Add/1 -> Divide/1
  r_stat/1 -> Bus Selector2/1, friction/4(r_stat)
  M_antr/1 -> friction/6(M_drive), Bus Selector1/1
  My/1 -> Bus Selector3/1
  Fl/1 -> friction/10(Fl), Bus Selector4/1
  Bus Selector3/1 -> Add/1  "<Ms_RF>"
  Bus Selector3/2 -> Add1/1  "<Ms_LF>"
  Bus Selector3/3 -> Add2/1  "<Ms_RR>"
  Bus Selector3/4 -> Add3/1  "<Ms_LR>"
  Divide/1 -> Bus Creator1/1, Discrete-Time Integrator2/1  "omegap_RF"
  Divide1/1 -> Bus Creator1/2, Discrete-Time Integrator1/1  "omegap_LF"
  Divide2/1 -> Bus Creator1/3, Discrete-Time Integrator3/1  "omegap_RR"
  Divide3/1 -> Bus Creator1/4, Discrete-Time Integrator4/1  "omegap_LR"
  Constant/1 -> Divide4/1, Divide5/1, Divide6/1, Divide7/1
  Divide4/1 -> Discrete-Time Integrator2/3
  Divide5/1 -> Discrete-Time Integrator1/3
  Divide6/1 -> Discrete-Time Integrator3/3
  Divide7/1 -> Discrete-Time Integrator4/3
  Unit Delay1/1 -> Divide4/2
  Unit Delay2/1 -> Divide5/2
  Unit Delay3/1 -> Divide6/2
  Unit Delay4/1 -> Divide7/2
  Product7/1 -> Add3/3
  [Iwf] -> Divide/2, Divide1/2
  M_brems/1 -> friction/5(M_brake), Bus Selector5/1
  Bus Selector1/1 -> Add4/1  "<M_antr_RF>"
  Bus Selector5/1 -> Add4/2  "<M_brems_RF>"
  Bus Selector1/2 -> Add5/1  "<M_antr_LF>"
  Bus Selector5/2 -> Add5/2  "<M_brems_LF>"
  Bus Selector1/3 -> Add6/1  "<M_antr_RR>"
  Bus Selector5/3 -> Add6/2  "<M_brems_RR>"
  Bus Selector1/4 -> Add7/1  "<M_antr_LR>"
  Bus Selector5/4 -> Add7/2  "<M_brems_LR>"
  r_dyn/1 -> Bus Selector6/1
  Bus Selector6/1 -> Unit Delay1/1  "<r_dyn_RF>"
  Bus Selector6/2 -> Unit Delay2/1  "<r_dyn_LF>"
  Bus Selector6/3 -> Unit Delay3/1  "<r_dyn_RR>"
  Bus Selector6/4 -> Unit Delay4/1  "<r_dyn_LR>"
  Fz/1 -> friction/1(Fz)
  Fs/1 -> friction/2(Fs)
  friction/1(M_fric_RF) -> Add/4
  friction/2(M_fric_LF) -> Add1/4
  friction/3(M_fric_RR) -> Add2/4
  friction/4(M_fric_LR) -> Add3/4
  delta/1 -> friction/7(delta)
  camber/1 -> friction/8(camber)
  z_wheel_body/1 -> friction/9(z_wheel_body)
  friction/5(fric_save) -> fric_save/1
  M_x/1 -> friction/11(M_x)
  M_z/1 -> friction/12(M_z)

== system vehicle_model/vehicle_model/wheel/calc_v ==
  delta : Inport
  beta : Inport  Port=2
  psi : Inport  Port=3
  v : Inport  Port=4
  calc_vl : Subsystem
  calc_vs : Subsystem
  vs : Outport  VectorParamsAs1DForOutWhenUnconnected=off
  vl : Outport  Port=2  VectorParamsAs1DForOutWhenUnconnected=off
  wires:
  calc_vs/1(vs) -> vs/1
  beta/1 -> calc_vs/7(beta), calc_vl/7(beta)
  v/1 -> calc_vs/5(v), calc_vl/5(v)
  calc_vl/1(vl) -> vl/1
  [lR] -> calc_vs/2(lR), calc_vl/2(lR)
  [lF] -> calc_vs/1(lF), calc_vl/1(lF)
  [sR05] -> calc_vs/4(sR05), calc_vl/4(sR05)
  [sF05] -> calc_vs/3(sF05), calc_vl/3(sF05)
  delta/1 -> calc_vs/8(delta), calc_vl/8(delta)
  psi/1 -> calc_vs/6(psi), calc_vl/6(psi)
  [ySP] -> calc_vl/9(ySP), calc_vs/9(ySP)

== system vehicle_model/vehicle_model/wheel/v0_korr ==
  vl : Inport
  r_dyn : Inport  Port=2
  omega : Inport  Port=3
  Bus Creator : BusCreator  Inputs=4
  Bus Selector : BusSelector  OutputSignals=vl_RF,vl_LF,vl_RR,vl_LR
  Bus Selector1 : BusSelector  OutputSignals=r_dyn_RF,r_dyn_LF,r_dyn_RR,r_dyn_LR
  Bus Selector2 : BusSelector  OutputSignals=omega_RF,omega_LF,omega_RR,omega_LR
  Subsystem1 : $bdroot/vehicle_model/wheel/v0_korr/Subsystem4  SystemSampleTime=-1  VariantActivationTime=update diagram  Latency=0  AutoFrameSizeCalculation=off
  Subsystem2 : $bdroot/vehicle_model/wheel/v0_korr/Subsystem4  SystemSampleTime=-1  VariantActivationTime=update diagram  Latency=0  AutoFrameSizeCalculation=off
  Subsystem3 : $bdroot/vehicle_model/wheel/v0_korr/Subsystem4  SystemSampleTime=-1  VariantActivationTime=update diagram  Latency=0  AutoFrameSizeCalculation=off
  Subsystem4 : Subsystem
  v_low : Constant  Value=0.01  VectorParams1D=off
  omega_out : Outport  VectorParamsAs1DForOutWhenUnconnected=off
  wires:
  Subsystem3/1 -> Bus Creator/4  "omega_LR"
  Subsystem2/1 -> Bus Creator/3  "omega_RR"
  Subsystem1/1 -> Bus Creator/2  "omega_LF"
  Subsystem4/1(omega_out) -> Bus Creator/1  "omega_RF"
  Bus Selector2/4 -> Subsystem3/4  "<omega_LR>"
  Bus Selector2/3 -> Subsystem2/4  "<omega_RR>"
  Bus Selector2/2 -> Subsystem1/4  "<omega_LF>"
  Bus Selector2/1 -> Subsystem4/4(omega)  "<omega_RF>"
  Bus Selector1/4 -> Subsystem3/3  "<r_dyn_LR>"
  Bus Selector1/3 -> Subsystem2/3  "<r_dyn_RR>"
  Bus Selector1/2 -> Subsystem1/3  "<r_dyn_LF>"
  Bus Selector1/1 -> Subsystem4/3(r_dyn)  "<r_dyn_RF>"
  v_low/1 -> Subsystem1/2, Subsystem2/2, Subsystem3/2, Subsystem4/2(v_low)
  Bus Selector/4 -> Subsystem3/1  "<vl_LR>"
  Bus Selector/3 -> Subsystem2/1  "<vl_RR>"
  Bus Selector/2 -> Subsystem1/1  "<vl_LF>"
  Bus Selector/1 -> Subsystem4/1(vl)  "<vl_RF>"
  Bus Creator/1 -> omega_out/1
  omega/1 -> Bus Selector2/1
  r_dyn/1 -> Bus Selector1/1
  vl/1 -> Bus Selector/1

== system vehicle_model/vehicle_model/wheel/wheel_lift ==
  Fz_spring : Inport
  Fz_tire_wheel : Inport  Port=2
  init_pos : Inport  Port=3
  Bus Selector : BusSelector  OutputSignals=Fz_tire_wheel_RF,Fz_tire_wheel_LF,Fz_tire_wheel_RR,Fz_tire_wheel_LR
  Bus Selector1 : BusSelector  OutputSignals=Fz_RF,Fz_LF,Fz_RR,Fz_LR
  Bus Selector2 : BusSelector  OutputSignals=zroad_RF0,zroad_LF0,zroad_RR0,zroad_LR0
  wheel_lift_LF : $bdroot/vehicle_model/wheel/wheel_lift/wheel_lift_RF  SystemSampleTime=-1  VariantActivationTime=update diagram  Latency=0  AutoFrameSizeCalculation=off
  wheel_lift_LR : $bdroot/vehicle_model/wheel/wheel_lift/wheel_lift_RR  SystemSampleTime=-1  VariantActivationTime=update diagram  Latency=0  AutoFrameSizeCalculation=off
  wheel_lift_RF : Subsystem
  wheel_lift_RR : Subsystem
  zwheel_RF : Outport  VectorParamsAs1DForOutWhenUnconnected=off
  zwheel_LF : Outport  Port=2  VectorParamsAs1DForOutWhenUnconnected=off
  zwheel_RR : Outport  Port=3  VectorParamsAs1DForOutWhenUnconnected=off
  zwheel_LR : Outport  Port=4  VectorParamsAs1DForOutWhenUnconnected=off
  wires:
  wheel_lift_RF/1(zwheel) -> zwheel_RF/1
  Fz_tire_wheel/1 -> Bus Selector/1
  wheel_lift_LF/1 -> zwheel_LF/1
  Fz_spring/1 -> Bus Selector1/1
  wheel_lift_RR/1(zwheel) -> zwheel_RR/1
  wheel_lift_LR/1 -> zwheel_LR/1
  Bus Selector/1 -> wheel_lift_RF/1(Fz_tire_wheel)  "<Fz_tire_wheel_RF>"
  Bus Selector/2 -> wheel_lift_LF/1  "<Fz_tire_wheel_LF>"
  Bus Selector/3 -> wheel_lift_RR/1(Fz_tire_wheel)  "<Fz_tire_wheel_RR>"
  Bus Selector/4 -> wheel_lift_LR/1  "<Fz_tire_wheel_LR>"
  Bus Selector1/2 -> wheel_lift_LF/2  "<Fz_LF>"
  Bus Selector1/1 -> wheel_lift_RF/2(Fzt)  "<Fz_RF>"
  Bus Selector1/3 -> wheel_lift_RR/2(Fzt)  "<Fz_RR>"
  Bus Selector1/4 -> wheel_lift_LR/2  "<Fz_LR>"
  init_pos/1 -> Bus Selector2/1
  Bus Selector2/1 -> wheel_lift_RF/3(z_init)  "<zroad_RF0>"
  Bus Selector2/2 -> wheel_lift_LF/3  "<zroad_LF0>"
  Bus Selector2/3 -> wheel_lift_RR/3(z_init)  "<zroad_RR0>"
  Bus Selector2/4 -> wheel_lift_LR/3  "<zroad_LR0>"

== system vehicle_model/simplified_vehicle_model/body_chassis_vert/horizontal/P_aer  ==
  P_aer_x : Inport
  Bus Creator1 : BusCreator  Inputs=3
  P_aer_y : Constant  Value=0
  P_aer_z : Constant  Value=0
  P_aer : Outport  VectorParamsAs1DForOutWhenUnconnected=off
  wires:
  P_aer_z/1 -> Bus Creator1/3  "P_aer_z"
  P_aer_y/1 -> Bus Creator1/2  "P_aer_y"
  P_aer_x/1 -> Bus Creator1/1  "P_aer_x"
  Bus Creator1/1 -> P_aer/1

== system vehicle_model/simplified_vehicle_model/body_chassis_vert/horizontal/acc ==
  Fl : Inport
  pitch : Inport  Port=2
  F_aer : Inport  Port=3
  Add : Sum  Inputs=++--
  Bus Selector : BusSelector  OutputSignals=Fl_F,Fl_R
  Divide : Product  Inputs=*/
  Gain : Gain  Gain=0.5
  Gain1 : Gain  Gain=0.5
  Product4 : Product  Inputs=3  RndMeth=Zero
  Trigonometric Function5 : Trigonometry
  a : Outport  VectorParamsAs1DForOutWhenUnconnected=off
  wires:
  Bus Selector/2 -> Add/2  "<Fl_R>"
  Bus Selector/1 -> Add/1  "<Fl_F>"
  Divide/1 -> a/1
  Fl/1 -> Bus Selector/1
  Add/1 -> Divide/1
  F_aer/1 -> Gain1/1
  [m] -> Gain/1
  Gain/1 -> Divide/2, Product4/3
  [g] -> Product4/2
  Trigonometric Function5/1 -> Product4/1
  pitch/1 -> Trigonometric Function5/1
  Product4/1 -> Add/4
  Gain1/1 -> Add/3

== system vehicle_model/simplified_vehicle_model/body_chassis_vert/horizontal/aerodynamics ==
  rho_air : Inport
  v : Inport  Port=2
  v_wind : Inport  Port=3
  Bus Selector2 : BusSelector  OutputSignals=vx
  Constant : Constant  Value=0.5
  Math Function2 : Math  Operator=square  SignedPower=on  SaturateOnIntegerOverflow=on
  Product{,1..2,4} (4 alike) : Product  RndMeth=Zero
  Sum5 : Sum  Inputs=++|
  Unary Minus : UnaryMinus
  F_aer : Outport  VectorParamsAs1DForOutWhenUnconnected=off
  wires:
  Constant/1 -> Product/1
  [cx] -> Product/2
  [Afront] -> Product1/1
  rho_air/1 -> Product1/2
  Product/1 -> Product2/1
  Product1/1 -> Product2/2
  Product2/1 -> Product4/2  "air_x"
  v_wind/1 -> Bus Selector2/1
  Bus Selector2/1 -> Sum5/2  "<vx>"
  Product4/1 -> F_aer/1  "F_aer_x"
  v/1 -> Unary Minus/1
  Math Function2/1 -> Product4/1
  Unary Minus/1 -> Sum5/1
  Sum5/1 -> Math Function2/1  "vx"

== system vehicle_model/simplified_vehicle_model/body_chassis_vert/suspension/damper ==
  note: Fz_damper is refered to wheel
  z_pitch : Inport
  z_body_vert : Inport  Port=2
  z_wheel_vert : Inport  Port=3
  Bus Creator : BusCreator  Inputs=2
  Bus Creator1 : BusCreator  Inputs=2
  Bus Selector1 : BusSelector  OutputSignals=z_pitch_Front.z_pitch_Fp,z_pitch_Rear.z_pitch_Rp
  Bus Selector2 : BusSelector  OutputSignals=z_vertp
  Bus Selector3 : BusSelector  OutputSignals=zwheel_F.zwheelp,zwheel_R.zwheelp
  Front : Subsystem
  Rear : Subsystem
  F_damper : Outport  VectorParamsAs1DForOutWhenUnconnected=off
  P_damper : Outport  Port=2  VectorParamsAs1DForOutWhenUnconnected=off
  wires:
  Rear/2(P_damper) -> Bus Creator1/2  "P_damper_Rear"
  Front/2(P_damper) -> Bus Creator1/1  "P_damper_Front"
  Bus Creator1/1 -> P_damper/1
  z_wheel_vert/1 -> Bus Selector3/1
  Bus Creator/1 -> F_damper/1
  z_pitch/1 -> Bus Selector1/1
  Rear/1(Fz_damper) -> Bus Creator/2  "Fz_damper_Rear"
  Front/1(Fz_damper) -> Bus Creator/1  "Fz_damper_Front"
  z_body_vert/1 -> Bus Selector2/1
  Bus Selector2/1 -> Rear/2(z_vertp), Front/2(z_vertp)  "<z_vertp>"
  Bus Selector1/2 -> Rear/1(z_pitchp)  "<z_pitch_Rp>"
  Bus Selector1/1 -> Front/1(z_pitchp)  "<z_pitch_Fp>"
  Bus Selector3/1 -> Front/3(z_wheel_vertp)  "<zwheelp>"
  Bus Selector3/2 -> Rear/3(z_wheel_vertp)  "<zwheelp>"

== system vehicle_model/simplified_vehicle_model/body_chassis_vert/suspension/spring ==
  note: Fz_spring is refered to wheel
  z_pitch : Inport
  z_vert : Inport  Port=2
  z_wheel_vert : Inport  Port=3
  Bus Creator : BusCreator  Inputs=2
  Bus Creator1 : BusCreator  Inputs=2
  Bus Selector1 : BusSelector  OutputSignals=z_pitch_Front.z_pitch_F,z_pitch_Rear.z_pitch_R
  Bus Selector2 : BusSelector  OutputSignals=z_vert
  Bus Selector3 : BusSelector  OutputSignals=zwheel_F.zwheel,zwheel_R.zwheel
  Front : Subsystem
  Rear : Subsystem
  Fz_spring : Outport  VectorParamsAs1DForOutWhenUnconnected=off
  z_wheel : Outport  Port=2  VectorParamsAs1DForOutWhenUnconnected=off
  wires:
  Bus Selector3/2 -> Rear/3(z_wheel_vert)  "<zwheel>"
  Front/1(Fz_spring) -> Bus Creator/1  "Fz_spring_Front"
  Rear/1(Fz_spring) -> Bus Creator/2  "Fz_spring_Rear"
  Bus Selector1/1 -> Front/1(z_pitch)  "<z_pitch_F>"
  Bus Creator/1 -> Fz_spring/1
  z_vert/1 -> Bus Selector2/1
  Bus Selector3/1 -> Front/3(z_wheel_vert)  "<zwheel>"
  z_wheel_vert/1 -> Bus Selector3/1
  Bus Selector2/1 -> Rear/2(z_vert), Front/2(z_vert)  "<z_vert>"
  Bus Creator1/1 -> z_wheel/1
  Front/2(z_wheel) -> Bus Creator1/1  "z_wheel_Front"
  Rear/2(z_wheel) -> Bus Creator1/2  "z_wheel_Rear"
  z_pitch/1 -> Bus Selector1/1
  Bus Selector1/2 -> Rear/1(z_pitch)  "<z_pitch_R>"

== system vehicle_model/simplified_vehicle_model/wheel/Tire_Model/mue ==
  "mue_road " : Inport
  Bus Selector6 : BusSelector  OutputSignals=mu_road_RF,mu_road_LF,mu_road_RR,mu_road_LR
  Gain : Gain  Gain=0.5
  Gain1 : Gain  Gain=0.5
  Sum : Sum
  Sum1 : Sum
  mue_road_front : Outport  VectorParamsAs1DForOutWhenUnconnected=off
  mue_road_rear : Outport  Port=2  VectorParamsAs1DForOutWhenUnconnected=off
  wires:
  Gain/1 -> mue_road_rear/1
  "mue_road "/1 -> Bus Selector6/1
  Bus Selector6/2 -> Sum1/2  "<mu_road_LF>"
  Bus Selector6/1 -> Sum1/1  "<mu_road_RF>"
  Sum/1 -> Gain/1
  Bus Selector6/3 -> Sum/1  "<mu_road_RR>"
  Bus Selector6/4 -> Sum/2  "<mu_road_LR>"
  Gain1/1 -> mue_road_front/1
  Sum1/1 -> Gain1/1

== system vehicle_model/simplified_vehicle_model/wheel/calc_omega/friction ==
  omega : Inport
  Begrenzung bei durchgehendem Rad : Subsystem
  Bus to Vector : BusToVector
  M_fric_F : Outport  VectorParamsAs1DForOutWhenUnconnected=off
  M_fric_R : Outport  Port=2  VectorParamsAs1DForOutWhenUnconnected=off
  wires:
  Begrenzung bei durchgehendem Rad/2(friction_R) -> M_fric_R/1
  Begrenzung bei durchgehendem Rad/1(friction_F) -> M_fric_F/1
  omega/1 -> Bus to Vector/1
  Bus to Vector/1 -> Begrenzung bei durchgehendem Rad/1(omega)

== system vehicle_model/simplified_vehicle_model/wheel/v0_korr/Subsystem1 ==
  vl : Inport
  v_low : Inport  Port=2
  r_dyn : Inport  Port=3
  omega : Inport  Port=4
  Abs : Abs
  Constant1 : Constant
  Constant2 : Constant  Value=pi
  Constant3 : Constant  Value=0.5
  Constant4 : Constant  Value=0  VectorParams1D=off
  Constant5 : Constant
  Divide1 : Product  Inputs=*/
  Divide2 : Product  Inputs=*/
  Divide{3..6} (4 alike) : Product  Inputs=**
  Gain : Gain  Gain=2
  Saturation Dynamic : simulink/Discontinuities/Saturation Dynamic  OutMin=[]  OutMax=[]  OutDataTypeStr=Inherit: Same as second input  OutDataType=fixdt(1, 16)  OutScaling=2^-10  DoSatur=off
  Saturation Dynamic1 : simulink/Discontinuities/Saturation Dynamic  OutMin=[]  OutMax=[]  OutDataTypeStr=Inherit: Same as second input  OutDataType=fixdt(1, 16)  OutScaling=2^-10  DoSatur=off
  Subtract : Sum  Inputs=+-
  Subtract1 : Sum
  Subtract2 : Sum  Inputs=-+
  Subtract3 : Sum  Inputs=+-
  Subtract5 : Sum
  Switch : Switch  Threshold=-0.0001
  Trigonometric Function : Trigonometry  Operator=cos
  omega_out : Outport  VectorParamsAs1DForOutWhenUnconnected=off
  wires:
  vl/1 -> Abs/1, Divide1/1
  Divide1/1 -> Divide5/2
  v_low/1 -> Subtract/2, Subtract3/2, Divide2/2, Saturation Dynamic/1, Gain/1
  r_dyn/1 -> Divide1/2
  Subtract/1 -> Switch/2
  Divide2/1 -> Divide3/1
  Constant2/1 -> Divide3/2
  Divide3/1 -> Trigonometric Function/1
  Trigonometric Function/1 -> Subtract1/1
  Constant1/1 -> Subtract1/2
  Subtract1/1 -> Divide4/1
  Constant3/1 -> Divide4/2
  Abs/1 -> Saturation Dynamic/2, Saturation Dynamic1/2
  Saturation Dynamic/1 -> Subtract/1
  Constant4/1 -> Saturation Dynamic1/3, Saturation Dynamic/3
  omega/1 -> Divide6/2
  Subtract5/1 -> omega_out/1
  Divide6/1 -> Subtract5/2
  Divide4/1 -> Switch/1
  Constant5/1 -> Switch/3, Subtract2/2
  Switch/1 -> Divide5/1, Subtract2/1
  Divide5/1 -> Subtract5/1
  Subtract2/1 -> Divide6/1
  Subtract3/1 -> Divide2/1
  Saturation Dynamic1/1 -> Subtract3/1
  Gain/1 -> Saturation Dynamic1/1

== system vehicle_model/simplified_vehicle_model/wheel/wheel_lift/wheel_lift_F ==
  Fz_tire_wheel : Inport
  Fzt : Inport  Port=2
  z_init_front : Inport  Port=3
  Add : Sum  Inputs=+-
  Bus Creator : BusCreator  Inputs=3
  Discrete-Time Integrator : DiscreteIntegrator  ExternalReset=level  SampleTime=-1  ICPrevOutput=DiscIntNeverNeededParam  ICPrevScaledInput=DiscIntNeverNeededParam
  Discrete-Time Integrator1 : DiscreteIntegrator  ExternalReset=level  InitialConditionSource=external  SampleTime=-1  ICPrevOutput=DiscIntNeverNeededParam  ICPrevScaledInput=DiscIntNeverNeededParam
  Divide : Product  Inputs=*/
  Gain : Gain  Gain=0.5
  zwheel_front : Outport  VectorParamsAs1DForOutWhenUnconnected=off
  wires:
  z_init_front/1 -> Discrete-Time Integrator1/3
  [reset] -> Discrete-Time Integrator1/2, Discrete-Time Integrator/2
  Gain/1 -> Divide/2
  [m_usF] -> Gain/1
  Bus Creator/1 -> zwheel_front/1
  Discrete-Time Integrator1/1 -> Bus Creator/1  "zwheel"
  Discrete-Time Integrator/1 -> Bus Creator/2, Discrete-Time Integrator1/1  "zwheelp"
  Divide/1 -> Bus Creator/3, Discrete-Time Integrator/1  "zwheelpp"
  Fzt/1 -> Add/2
  Fz_tire_wheel/1 -> Add/1
  Add/1 -> Divide/1

== system vehicle_model/simplified_vehicle_model/wheel/wheel_lift/wheel_lift_R ==
  Fz_tire_wheel : Inport
  Fzt : Inport  Port=2
  z_init_rear : Inport  Port=3
  Add : Sum  Inputs=+-
  Bus Creator : BusCreator  Inputs=3
  Discrete-Time Integrator : DiscreteIntegrator  ExternalReset=level  SampleTime=-1  ICPrevOutput=DiscIntNeverNeededParam  ICPrevScaledInput=DiscIntNeverNeededParam
  Discrete-Time Integrator1 : DiscreteIntegrator  ExternalReset=level  InitialConditionSource=external  SampleTime=-1  ICPrevOutput=DiscIntNeverNeededParam  ICPrevScaledInput=DiscIntNeverNeededParam
  Divide : Product  Inputs=*/
  Gain : Gain  Gain=0.5
  zwheel_rear : Outport  VectorParamsAs1DForOutWhenUnconnected=off
  wires:
  z_init_rear/1 -> Discrete-Time Integrator1/3
  [reset] -> Discrete-Time Integrator1/2, Discrete-Time Integrator/2
  Gain/1 -> Divide/2
  [m_usR] -> Gain/1
  Bus Creator/1 -> zwheel_rear/1
  Discrete-Time Integrator1/1 -> Bus Creator/1  "zwheel"
  Discrete-Time Integrator/1 -> Bus Creator/2, Discrete-Time Integrator1/1  "zwheelp"
  Divide/1 -> Bus Creator/3, Discrete-Time Integrator/1  "zwheelpp"
  Fzt/1 -> Add/2
  Fz_tire_wheel/1 -> Add/1
  Add/1 -> Divide/1

== system vehicle_model/simplified_vehicle_model/wheel/wheel_lift/zroad ==
  init_pos : Inport
  Bus Selector6 : BusSelector  OutputSignals=zroad_RF0,zroad_LF0,zroad_RR0,zroad_LR0
  Gain : Gain  Gain=0.5
  Gain1 : Gain  Gain=0.5
  Sum : Sum
  Sum1 : Sum
  zroad_front : Outport  VectorParamsAs1DForOutWhenUnconnected=off
  zroad_rear : Outport  Port=2  VectorParamsAs1DForOutWhenUnconnected=off
  wires:
  Gain/1 -> zroad_rear/1
  init_pos/1 -> Bus Selector6/1
  Bus Selector6/2 -> Sum1/2  "<zroad_LF0>"
  Bus Selector6/1 -> Sum1/1  "<zroad_RF0>"
  Sum/1 -> Gain/1
  Bus Selector6/3 -> Sum/1  "<zroad_RR0>"
  Bus Selector6/4 -> Sum/2  "<zroad_LR0>"
  Gain1/1 -> zroad_front/1
  Sum1/1 -> Gain1/1
